simulink model "identification"  (R2017a)
settings: Solver=ode1  StartTime=0  StopTime=125  FixedStep=0.1  RelTol=1e-3  EnableMultiTasking=on
StartFcn:
  | initialize
values from neighbouring files (symbols this model uses):
  ad = Td/(Td + N*T0)    (= 0.994807351258)    [model_params.m]
  b = 0.2352    [model_params.m]
  bd = Kp*Td*N/(Td + N*T0)    (= 0.312545231066)    [model_params.m]
  bi1 = Kp*T0/Ti    (= 0.0654877697842)    [model_params.m]
  c = 0.7181    [model_params.m]
  GAMAin = 100    [model_params.m]
  Kp = K1(2:4)    [dlqr_reg.m]    (also in model_params.m = 0.6502)
  Ks = 0.012    [model_params.m]
  MUmax = 0.55    [model_params.m]
  T0 = 0.0056    [dlqr_reg.m]    (also in model_params.m)
  Ysx = 0.5    [model_params.m]
settings Model: Creator=Alex  LastModifiedBy=user
settings DataIOCC: LimitDataPoints=on  SaveFormat=Array  SignalLoggingSaveFormat=ModelDataLogs
settings OptimizationCC: LifeSpan=inf
settings DebuggingCC: UnderspecifiedInitializationDetection=Classic  MergeDetectMultiDrivingBlocksExec=none  SolverPrmCheckMsg=warning  FcnCallInpInsideContextMsg=warning  StateNameClashWarn=warning  SFUnexpectedBacktrackingDiag=warning  SFNoUnconditionalDefaultTransitionDiag=warning  SFExecutionAtInitializationDiag=none
settings HardwareCC: ProdBitPerPointer=32  ProdBitPerSizeT=32  ProdBitPerPtrDiffT=32  ProdLargestAtomicFloat=None  ProdIntDivRoundTo=Undefined  ProdEndianess=Unspecified  ProdWordSize=32  ProdHWDeviceType=32-bit Generic
settings ModelReferenceCC: PropagateSignalLabelsOutOfModel=off
settings GRTTargetCC: TargetLangStandard=C89/C90 (ANSI)  GeneratePreprocessorConditionals=Disable all  CombineOutputUpdateFcns=off  GRTInterface=on
settings ConfigComp: CovMetricSettings=dw  CovHtmlReporting=on  CovSaveCumulativeToWorkspaceVar=on  CovSaveSingleToWorkspaceVar=on  CovExternalEMLEnable=off

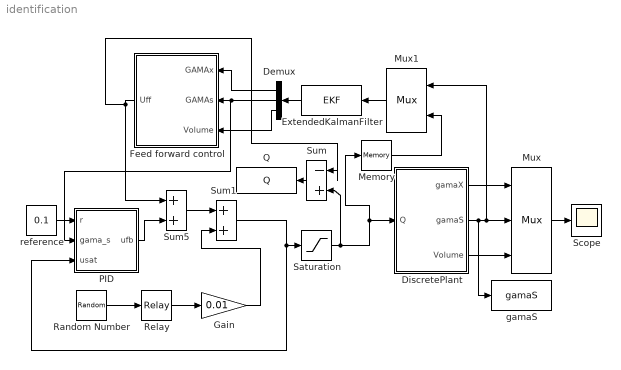
== system identification ==
  Demux : Demux  Outputs=3
  DiscretePlant : Subsystem
  ExtendedKalmanFilter : MATLABFcn  MATLABFcn=EKF  OutputDimensions=3  Output1D=off
  Feed forward control : Subsystem
  Gain : Gain  Gain=0.01  SampleTime=0.1
  Memory : Memory
  Mux : Mux  Inputs=3
      settings: DisplayOption=signals
  Mux1 : Mux  Inputs=2
      settings: DisplayOption=signals
  PID : Subsystem
  Q : ToWorkspace  VariableName=Q  SaveFormat=Timeseries  SampleTime=-1
  Random Number : RandomNumber  Seed=24334  SampleTime=0.1
  Relay : Relay  OnOutputValue=0.2  OffOutputValue=-0.2
  Saturation : Saturate  UpperLimit=1  LowerLimit=0
  Scope : Scope
  Sum : Sum  Inputs=|-+
  Sum1 : Sum
  Sum5 : Sum
  "gamaS " : ToWorkspace  VariableName=gamaS  SaveFormat=Timeseries  SampleTime=-1
  reference : Constant  Value=0.1
  wires:
  PID/1(ufb) -> Sum5/2
  reference/1 -> PID/1(r)
  Saturation/1 -> Sum/2, Memory/1, DiscretePlant/1(Q)
  Feed forward control/1(Uff) -> Sum5/1, Sum/1
  DiscretePlant/2(gamaS) -> "gamaS "/1, Mux/2, Mux1/1
  Mux1/1 -> ExtendedKalmanFilter/1
  Memory/1 -> Mux1/2
  Random Number/1 -> Relay/1
  Sum1/1 -> PID/3(usat), Saturation/1
  Sum5/1 -> Sum1/1
  Relay/1 -> Gain/1
  Gain/1 -> Sum1/2
  DiscretePlant/1(gamaX) -> Mux/1
  DiscretePlant/3(Volume) -> Mux/3
  ExtendedKalmanFilter/1 -> Demux/1
  Demux/1 -> Feed forward control/1(GAMAx)
  Demux/2 -> Feed forward control/2(GAMAs), PID/2(gama_s)
  Demux/3 -> Feed forward control/3(Volume)
  Mux/1 -> Scope/1
  Sum/1 -> Q/1

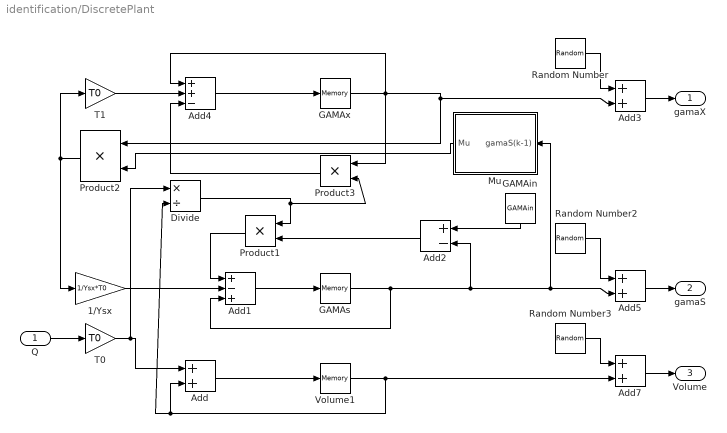
== system identification/DiscretePlant ==
  Q : Inport
  1/Ysx : Gain  Gain=1/Ysx*T0
  Add{,3,5,7} (4 alike) : Sum
  Add1 : Sum  Inputs=+-+
  Add2 : Sum  Inputs=+-
  Add4 : Sum  Inputs=++-
  Divide : Product  Inputs=*/
  GAMAin : Constant  Value=GAMAin
  GAMAs : Memory  X0=0.81
  GAMAx : Memory  X0=1.25
  Mu : Subsystem
  Product1 : Product  RndMeth=Zero
  Product2 : Product  RndMeth=Zero
  Product3 : Product  RndMeth=Zero
  Random Number : RandomNumber  Variance=0.0001  Seed=34645  SampleTime=0.1
  Random Number2 : RandomNumber  Variance=0.001  Seed=454645  SampleTime=0.1
  Random Number3 : RandomNumber  Variance=0.0001  Seed=4546  SampleTime=0.1
  T0 : Gain  Gain=T0
  T1 : Gain  Gain=T0
  Volume1 : Memory  X0=1.35
  gamaX : Outport
  gamaS : Outport  Port=2
  Volume : Outport  Port=3
  wires:
  Product1/1 -> Add1/1
  Add2/1 -> Product1/2
  GAMAin/1 -> Add2/1
  1/Ysx/1 -> Add1/2
  Product2/1 -> 1/Ysx/1, T1/1
  Product3/1 -> Add4/3
  Add1/1 -> GAMAs/1
  Add4/1 -> GAMAx/1
  Mu/1(Mu) -> Product2/2
  GAMAs/1 -> Add2/2, Mu/1(gamaS(k-1)), Add5/2, Add1/3
  GAMAx/1 -> Product3/1, Add4/1, Product2/1, Add3/2
  Add/1 -> Volume1/1
  Volume1/1 -> Divide/2, Add/2, Add7/2
  T0/1 -> Add/1, Divide/1
  Divide/1 -> Product1/1, Product3/2
  T1/1 -> Add4/2
  Random Number/1 -> Add3/1
  Add3/1 -> gamaX/1
  Random Number2/1 -> Add5/1
  Add5/1 -> gamaS/1
  Random Number3/1 -> Add7/1
  Q/1 -> T0/1
  Add7/1 -> Volume/1

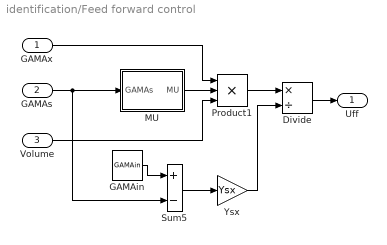
== system identification/Feed forward control ==
  GAMAx : Inport
  GAMAs : Inport  Port=2
  Volume : Inport  Port=3
  Divide : Product  Inputs=*/
  GAMAin : Constant  Value=GAMAin
  MU : Subsystem
  Product1 : Product  Inputs=3  RndMeth=Zero
  Sum5 : Sum  Inputs=+-
  Ysx : Gain  Gain=Ysx
  Uff : Outport
  wires:
  GAMAs/1 -> MU/1(GAMAs), Sum5/2
  GAMAx/1 -> Product1/1
  MU/1(MU) -> Product1/2
  Volume/1 -> Product1/3
  Sum5/1 -> Ysx/1
  GAMAin/1 -> Sum5/1
  Product1/1 -> Divide/1
  Ysx/1 -> Divide/2
  Divide/1 -> Uff/1

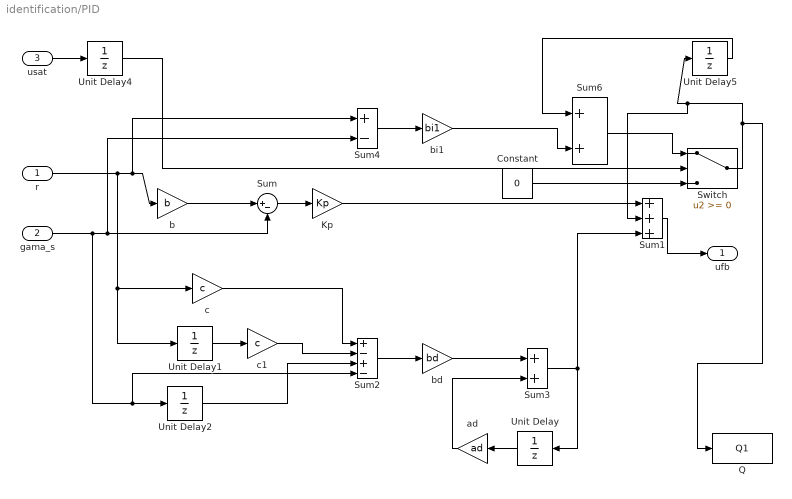
== system identification/PID ==
  r : Inport
  gama_s : Inport  Port=2
  usat : Inport  Port=3
  Constant : Constant  Value=0
  Kp : Gain  Gain=Kp
  Q : ToWorkspace  VariableName=Q1  SampleTime=-1
  Sum : Sum  Inputs=|+-
  Sum1 : Sum  Inputs=+++
  Sum2 : Sum  Inputs=+-+-
  Sum3 : Sum
  Sum4 : Sum  Inputs=+-
  Sum6 : Sum
  Switch : Switch
  Unit Delay{,1..2,4..5} (5 alike) : UnitDelay  SampleTime=-1
  ad : Gain  Gain=ad
  b : Gain  Gain=b
  bd : Gain  Gain=bd
  bi1 : Gain  Gain=bi1
  c : Gain  Gain=c
  c1 : Gain  Gain=c
  ufb : Outport
  wires:
  Sum6/1 -> Switch/1
  bi1/1 -> Sum6/2
  Sum4/1 -> bi1/1
  Kp/1 -> Sum1/1
  Sum1/1 -> ufb/1
  Sum3/1 -> Sum1/3, Unit Delay/1
  bd/1 -> Sum3/1
  ad/1 -> Sum3/2
  Sum2/1 -> bd/1
  c1/1 -> Sum2/2
  c/1 -> Sum2/1
  Unit Delay2/1 -> Sum2/3
  Unit Delay1/1 -> c1/1
  Unit Delay/1 -> ad/1
  Sum/1 -> Kp/1
  gama_s/1 -> Sum/2, Sum4/2, Sum2/4, Unit Delay2/1
  b/1 -> Sum/1
  r/1 -> Sum4/1, b/1, Unit Delay1/1, c/1
  usat/1 -> Unit Delay4/1
  Constant/1 -> Switch/3
  Unit Delay4/1 -> Switch/2
  Switch/1 -> Unit Delay5/1, Sum1/2, Q/1
  Unit Delay5/1 -> Sum6/1

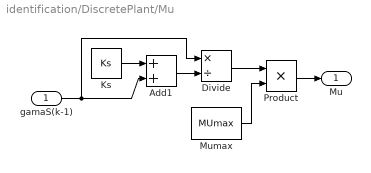
== system identification/DiscretePlant/Mu ==
  gamaS(k-1) : Inport
  Add1 : Sum
  Divide : Product  Inputs=*/
  Ks : Constant  Value=Ks
  Mumax : Constant  Value=MUmax
  Product : Product  RndMeth=Zero
  Mu : Outport
  wires:
  Ks/1 -> Add1/1
  Add1/1 -> Divide/2
  Divide/1 -> Product/1
  Mumax/1 -> Product/2
  Product/1 -> Mu/1
  gamaS(k-1)/1 -> Add1/2, Divide/1

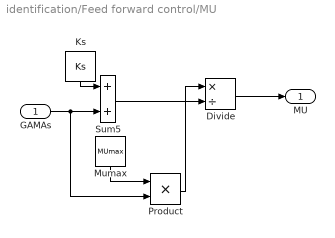
== system identification/Feed forward control/MU ==
  GAMAs : Inport
  Divide : Product  Inputs=*/
  Ks : Constant  Value=Ks
  Mumax : Constant  Value=MUmax
  Product : Product  RndMeth=Zero
  Sum5 : Sum
  MU : Outport
  wires:
  Product/1 -> Divide/1
  Mumax/1 -> Product/1
  Sum5/1 -> Divide/2
  GAMAs/1 -> Sum5/2, Product/2
  Ks/1 -> Sum5/1
  Divide/1 -> MU/1
